simulink library "Quaternion_Multiplication"  (R2016a)
settings: Solver=ode45  StartTime=0.0  StopTime=10.0  RelTol=1e-3
settings Model: Creator=devantormey  LastModifiedBy=devantormey
settings DataIOCC: LimitDataPoints=on
settings DebuggingCC: AllowSymbolicDim=off

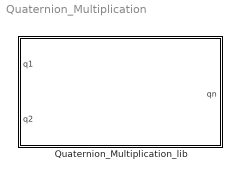
== system Quaternion_Multiplication ==
  Quaternion_Multiplication_lib : Subsystem

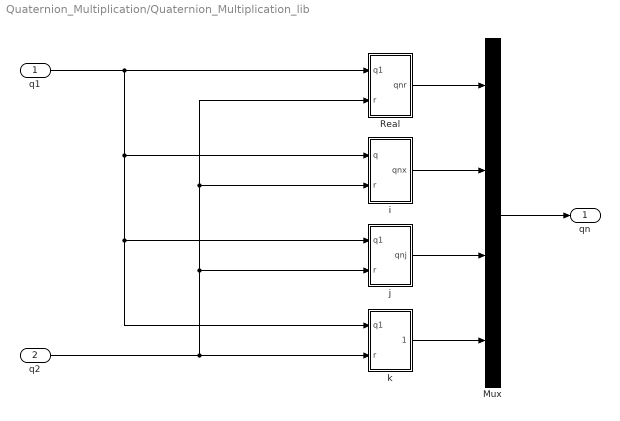
== system Quaternion_Multiplication/Quaternion_Multiplication_lib ==
  "q1 " : Inport
  q2 : Inport  Port=2
  Mux : Mux
  Real : Subsystem
  i : Subsystem
  j : Subsystem
  k : Subsystem
  qn : Outport
  wires:
  Mux/1 -> qn/1
  "q1 "/1 -> j/1(q1), k/1(q1), i/1(q), Real/1("q1 ")
  q2/1 -> k/2(r), j/2(r), Real/2(r), i/2(r)
  Real/1("qnr ") -> Mux/1
  i/1(qnx) -> Mux/2
  j/1(qnj) -> Mux/3
  k/1(qnk) -> Mux/4

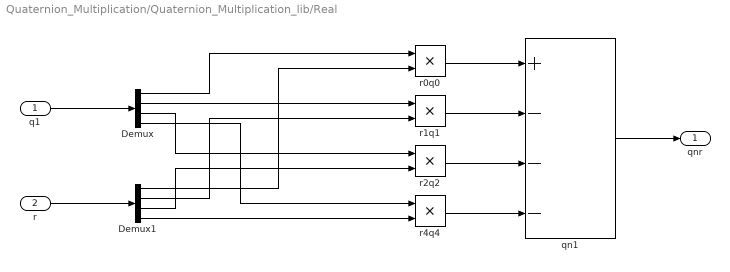
== system Quaternion_Multiplication/Quaternion_Multiplication_lib/Real ==
  "q1 " : Inport
  r : Inport  Port=2
  Demux : Demux
  Demux1 : Demux
  qn1 : Sum  Inputs=+---
  r0q0 : Product
  r1q1 : Product
  r2q2 : Product
  r4q4 : Product
  "qnr " : Outport
  wires:
  r1q1/1 -> qn1/2
  r/1 -> Demux1/1
  qn1/1 -> "qnr "/1
  "q1 "/1 -> Demux/1
  r4q4/1 -> qn1/4
  r2q2/1 -> qn1/3
  r0q0/1 -> qn1/1
  Demux1/1 -> r0q0/2
  Demux/1 -> r0q0/1
  Demux1/2 -> r1q1/2
  Demux/2 -> r1q1/1
  Demux/3 -> r2q2/1
  Demux1/3 -> r2q2/2
  Demux1/4 -> r4q4/2
  Demux/4 -> r4q4/1

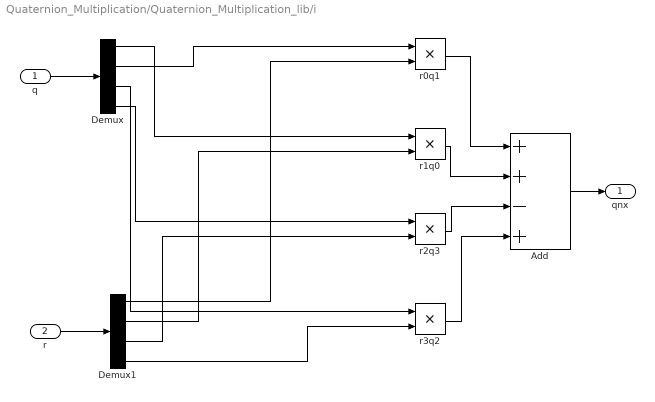
== system Quaternion_Multiplication/Quaternion_Multiplication_lib/i ==
  q : Inport
  r : Inport  Port=2
  Add : Sum  Inputs=++-+
  Demux : Demux
  Demux1 : Demux
  r0q1 : Product
  r1q0 : Product
  r2q3 : Product
  r3q2 : Product
  qnx : Outport
  wires:
  q/1 -> Demux/1
  r/1 -> Demux1/1
  Demux1/1 -> r0q1/2
  Demux/2 -> r0q1/1
  Demux1/2 -> r1q0/2
  Demux/1 -> r1q0/1
  Demux1/3 -> r2q3/2
  Demux1/4 -> r3q2/2
  Demux/4 -> r2q3/1
  Demux/3 -> r3q2/1
  Add/1 -> qnx/1
  r0q1/1 -> Add/1
  r1q0/1 -> Add/2
  r2q3/1 -> Add/3
  r3q2/1 -> Add/4

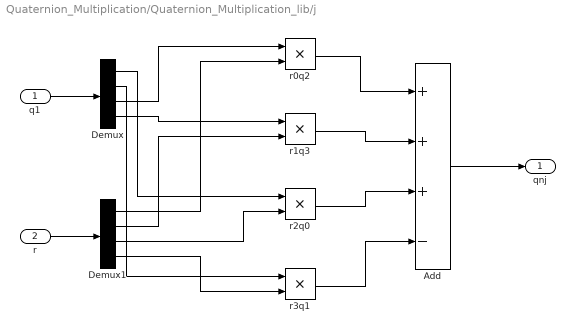
== system Quaternion_Multiplication/Quaternion_Multiplication_lib/j ==
  q1 : Inport
  r : Inport  Port=2
  Add : Sum  Inputs=+++-
  Demux : Demux
  Demux1 : Demux
  r0q2 : Product
  r1q3 : Product
  r2q0 : Product
  r3q1 : Product
  qnj : Outport
  wires:
  r/1 -> Demux1/1
  q1/1 -> Demux/1
  Demux1/1 -> r0q2/2
  Demux/3 -> r0q2/1
  Demux1/2 -> r1q3/2
  Demux/4 -> r1q3/1
  Demux1/3 -> r2q0/2
  Demux/1 -> r2q0/1
  Demux1/4 -> r3q1/2
  Demux/2 -> r3q1/1
  Add/1 -> qnj/1
  r0q2/1 -> Add/1
  r1q3/1 -> Add/2
  r2q0/1 -> Add/3
  r3q1/1 -> Add/4

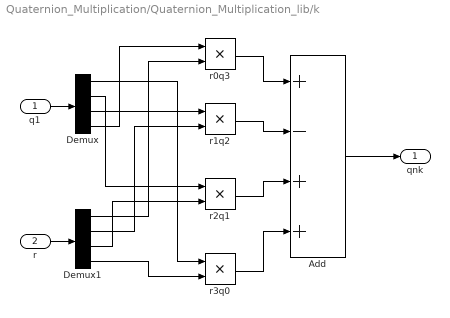
== system Quaternion_Multiplication/Quaternion_Multiplication_lib/k ==
  q1 : Inport
  r : Inport  Port=2
  Add : Sum  Inputs=+-++
  Demux : Demux
  Demux1 : Demux
  r0q3 : Product
  r1q2 : Product
  r2q1 : Product
  r3q0 : Product
  qnk : Outport
  wires:
  r/1 -> Demux1/1
  q1/1 -> Demux/1
  Demux1/1 -> r0q3/2
  Demux/4 -> r0q3/1
  Demux1/2 -> r1q2/2
  Demux/3 -> r1q2/1
  Demux1/3 -> r2q1/2
  Demux/2 -> r2q1/1
  Demux1/4 -> r3q0/2
  Demux/1 -> r3q0/1
  r0q3/1 -> Add/1
  r1q2/1 -> Add/2
  r2q1/1 -> Add/3
  r3q0/1 -> Add/4
  Add/1 -> qnk/1
